simulink model "MassTransfer"  (R2023a)
settings: Solver=ode4  StartTime=0.0  StopTime=7540  FixedStep=Delta  RelTol=1e-3
values from neighbouring files (symbols this model uses):
  C2Ini = 1.6    [MassTransferModelData.m]
  C3Ini = 0    [MassTransferModelData.m]
  C4Ini = 0    [MassTransferModelData.m]
  C5Ini = 1.6    [MassTransferModelData.m]
  Delta = 5    [MassTransferModelData.m]
  F = 96485    [MassTransferModelData.m]
  NCells = 120    [MassTransferModelData.m]
  VCell = 0.4968    [MassTransferModelData.m]
  VTank = 500    [MassTransferModelData.m]
  z = 1    [MassTransferModelData.m]
undefined symbols (not defined in the file or in its folder): DiscIntNeverNeededParam
(part 2 of 3)

== system MassTransfer/Liibrary block/simulink blocks/C2Cell ==
  QCell : Inport
  CTank : Inport  Port=2
  I : Inport  Port=3
  Constant : Constant  Value=F
  Constant1 : Constant  Value=VCell
  Constant2 : Constant  Value=2
  Discrete-Time Integrator : DiscreteIntegrator  IntegratorMethod=Integration: Backward Euler  InitialCondition=C2Ini  SampleTime=-1  ICPrevOutput=DiscIntNeverNeededParam  ICPrevScaledInput=DiscIntNeverNeededParam
  Divide : Product  Inputs=*/
  Divide1 : Product  Inputs=*/
  Gain : Gain  Gain=z
  Product : Product
  Product1 : Product
  Sum : Sum  Inputs=|+-
  Sum1 : Sum  Inputs=|+-
  CCell : Outport
  wires:
  I/1 -> Divide/1
  Constant/1 -> Gain/1
  Gain/1 -> Divide/2
  Constant1/1 -> Divide1/2
  Constant2/1 -> Divide1/1
  CTank/1 -> Sum/1
  Sum/1 -> Product/2
  QCell/1 -> Product/1
  Product/1 -> Sum1/1
  Divide/1 -> Sum1/2
  Sum1/1 -> Product1/1
  Divide1/1 -> Product1/2
  Product1/1 -> Discrete-Time Integrator/1
  Discrete-Time Integrator/1 -> Sum/2, CCell/1

== system MassTransfer/Liibrary block/simulink blocks/C2Tank ==
  QTank : Inport
  CCell : Inport  Port=2
  Constant : Constant  Value=VTank
  Discrete-Time Integrator : DiscreteIntegrator  IntegratorMethod=Integration: Backward Euler  InitialCondition=C2Ini  SampleTime=-1  ICPrevOutput=DiscIntNeverNeededParam  ICPrevScaledInput=DiscIntNeverNeededParam
  Divide : Product  Inputs=*/
  Product : Product
  Scope4 : Scope
  Sum : Sum  Inputs=|+-
  CTank : Outport
  wires:
  CCell/1 -> Sum/1, Scope4/1
  Sum/1 -> Product/1
  QTank/1 -> Divide/1
  Constant/1 -> Divide/2
  Divide/1 -> Product/2
  Product/1 -> Discrete-Time Integrator/1
  Discrete-Time Integrator/1 -> Sum/2, CTank/1

== system MassTransfer/Liibrary block/simulink blocks/C3Cell ==
  QCell : Inport
  CTank : Inport  Port=2
  I : Inport  Port=3
  Constant : Constant  Value=F
  Constant1 : Constant  Value=VCell
  Constant2 : Constant  Value=2
  Discrete-Time Integrator : DiscreteIntegrator  IntegratorMethod=Integration: Backward Euler  InitialCondition=C3Ini  SampleTime=-1  ICPrevOutput=DiscIntNeverNeededParam  ICPrevScaledInput=DiscIntNeverNeededParam
  Divide : Product  Inputs=*/
  Divide1 : Product  Inputs=*/
  Gain : Gain  Gain=z
  Product : Product
  Product1 : Product
  Sum : Sum  Inputs=|+-
  Sum1 : Sum  Inputs=|++
  CCell : Outport
  wires:
  Product1/1 -> Discrete-Time Integrator/1
  Divide1/1 -> Product1/2
  Sum1/1 -> Product1/1
  Divide/1 -> Sum1/2
  Product/1 -> Sum1/1
  QCell/1 -> Product/1
  Sum/1 -> Product/2
  CTank/1 -> Sum/1
  Constant2/1 -> Divide1/1
  Constant1/1 -> Divide1/2
  Gain/1 -> Divide/2
  Constant/1 -> Gain/1
  I/1 -> Divide/1
  Discrete-Time Integrator/1 -> Sum/2, CCell/1

== system MassTransfer/Liibrary block/simulink blocks/C3Tank ==
  QTank : Inport
  CCell : Inport  Port=2
  Constant : Constant  Value=VTank
  Discrete-Time Integrator : DiscreteIntegrator  IntegratorMethod=Integration: Backward Euler  InitialCondition=C3Ini  SampleTime=-1  ICPrevOutput=DiscIntNeverNeededParam  ICPrevScaledInput=DiscIntNeverNeededParam
  Divide : Product  Inputs=*/
  Product : Product
  Sum : Sum  Inputs=|+-
  CTank : Outport
  wires:
  Product/1 -> Discrete-Time Integrator/1
  Divide/1 -> Product/2
  Constant/1 -> Divide/2
  QTank/1 -> Divide/1
  Sum/1 -> Product/1
  CCell/1 -> Sum/1
  Discrete-Time Integrator/1 -> Sum/2, CTank/1

== system MassTransfer/Liibrary block/simulink blocks/C4Cell ==
  QCell : Inport
  CTank : Inport  Port=2
  I : Inport  Port=3
  Constant : Constant  Value=F
  Constant1 : Constant  Value=VCell
  Constant2 : Constant  Value=2
  Discrete-Time Integrator : DiscreteIntegrator  IntegratorMethod=Integration: Backward Euler  InitialCondition=C4Ini  SampleTime=-1  ICPrevOutput=DiscIntNeverNeededParam  ICPrevScaledInput=DiscIntNeverNeededParam
  Divide : Product  Inputs=*/
  Divide1 : Product  Inputs=*/
  Gain : Gain  Gain=z
  Product : Product
  Product1 : Product
  Sum : Sum  Inputs=|+-
  Sum1 : Sum  Inputs=|++
  CCell : Outport
  wires:
  I/1 -> Divide/1
  Constant/1 -> Gain/1
  Gain/1 -> Divide/2
  Constant1/1 -> Divide1/2
  Constant2/1 -> Divide1/1
  CTank/1 -> Sum/1
  Sum/1 -> Product/2
  QCell/1 -> Product/1
  Product/1 -> Sum1/1
  Divide/1 -> Sum1/2
  Sum1/1 -> Product1/1
  Divide1/1 -> Product1/2
  Product1/1 -> Discrete-Time Integrator/1
  Discrete-Time Integrator/1 -> Sum/2, CCell/1

== system MassTransfer/Liibrary block/simulink blocks/C4Tank ==
  QTank : Inport
  CCell : Inport  Port=2
  Constant : Constant  Value=VTank
  Discrete-Time Integrator : DiscreteIntegrator  IntegratorMethod=Integration: Backward Euler  InitialCondition=C4Ini  SampleTime=-1  ICPrevOutput=DiscIntNeverNeededParam  ICPrevScaledInput=DiscIntNeverNeededParam
  Divide : Product  Inputs=*/
  Product : Product
  Sum : Sum  Inputs=|+-
  CTank : Outport
  wires:
  CCell/1 -> Sum/1
  Sum/1 -> Product/1
  QTank/1 -> Divide/1
  Constant/1 -> Divide/2
  Divide/1 -> Product/2
  Product/1 -> Discrete-Time Integrator/1
  Discrete-Time Integrator/1 -> Sum/2, CTank/1

== system MassTransfer/Liibrary block/simulink blocks/C5Cell ==
  QCell : Inport
  CTank : Inport  Port=2
  I : Inport  Port=3
  Constant : Constant  Value=F
  Constant1 : Constant  Value=VCell
  Constant2 : Constant  Value=2
  Discrete-Time Integrator : DiscreteIntegrator  IntegratorMethod=Integration: Backward Euler  InitialCondition=C5Ini  SampleTime=-1  ICPrevOutput=DiscIntNeverNeededParam  ICPrevScaledInput=DiscIntNeverNeededParam
  Divide : Product  Inputs=*/
  Divide1 : Product  Inputs=*/
  Gain : Gain  Gain=z
  Product : Product
  Product1 : Product
  Sum : Sum  Inputs=|+-
  Sum1 : Sum  Inputs=|+-
  CCell : Outport
  wires:
  Product1/1 -> Discrete-Time Integrator/1
  Divide1/1 -> Product1/2
  Sum1/1 -> Product1/1
  Divide/1 -> Sum1/2
  Product/1 -> Sum1/1
  QCell/1 -> Product/1
  Sum/1 -> Product/2
  CTank/1 -> Sum/1
  Constant2/1 -> Divide1/1
  Constant1/1 -> Divide1/2
  Gain/1 -> Divide/2
  Constant/1 -> Gain/1
  I/1 -> Divide/1
  Discrete-Time Integrator/1 -> Sum/2, CCell/1

== system MassTransfer/Liibrary block/simulink blocks/C5Tank ==
  QTank : Inport
  CCell : Inport  Port=2
  Constant : Constant  Value=VTank
  Discrete-Time Integrator : DiscreteIntegrator  IntegratorMethod=Integration: Backward Euler  InitialCondition=C5Ini  SampleTime=-1  ICPrevOutput=DiscIntNeverNeededParam  ICPrevScaledInput=DiscIntNeverNeededParam
  Divide : Product  Inputs=*/
  Product : Product
  Sum : Sum  Inputs=|+-
  CTank : Outport
  wires:
  Product/1 -> Discrete-Time Integrator/1
  Divide/1 -> Product/2
  Constant/1 -> Divide/2
  QTank/1 -> Divide/1
  Sum/1 -> Product/1
  CCell/1 -> Sum/1
  Discrete-Time Integrator/1 -> Sum/2, CTank/1

== system MassTransfer/QF tests/Analitical/C2Cell ==
  QCell : Inport
  CTank : Inport  Port=2
  It : Inport  Port=3
  Constant : Constant  Value=-1
  Constant1 : Constant  Value=Delta
  Constant2 : Constant
  Constant3 : Constant  Value=F
  Constant4 : Constant  Value=VCell
  MATLAB Function : MATLAB Function  TreatAsAtomicUnit=on
  Memory : Memory  InitialCondition=C2Ini
  CCell : Outport
  wires:
  Constant/1 -> MATLAB Function/8(Sign)
  Constant1/1 -> MATLAB Function/9(Delta)
  Constant2/1 -> MATLAB Function/7(Z)
  QCell/1 -> MATLAB Function/1(QCell)
  Constant3/1 -> MATLAB Function/6(F)
  Constant4/1 -> MATLAB Function/4(VCell)
  MATLAB Function/1(CCell) -> Memory/1, CCell/1
  Memory/1 -> MATLAB Function/3(CCellAnt)
  It/1 -> MATLAB Function/5(It)
  CTank/1 -> MATLAB Function/2(CTank)

== system MassTransfer/QF tests/Analitical/C2Tank ==
  QTank : Inport
  CCell : Inport  Port=2
  Constant : Constant  Value=Delta
  Constant1 : Constant  Value=VTank
  MATLAB Function : MATLAB Function  TreatAsAtomicUnit=on
  Memory : Memory  InitialCondition=C2Ini
  Scope4 : Scope
  CTank : Outport
  wires:
  Constant/1 -> MATLAB Function/5(Delta)
  Constant1/1 -> MATLAB Function/4(VTank)
  MATLAB Function/1(CTank) -> Memory/1, CTank/1
  Memory/1 -> MATLAB Function/3(CTankAnt)
  QTank/1 -> MATLAB Function/1(Q)
  CCell/1 -> Scope4/1, MATLAB Function/2(CCell)

== system MassTransfer/QF tests/Analitical/C3Cell ==
  QCell : Inport
  CTank : Inport  Port=2
  It : Inport  Port=3
  Constant : Constant
  Constant1 : Constant  Value=Delta
  Constant2 : Constant
  Constant3 : Constant  Value=F
  Constant4 : Constant  Value=VCell
  MATLAB Function : MATLAB Function  TreatAsAtomicUnit=on
  Memory : Memory  InitialCondition=C3Ini
  CCell : Outport
  wires:
  It/1 -> MATLAB Function/5(It)
  Memory/1 -> MATLAB Function/3(CCellAnt)
  MATLAB Function/1(CCell) -> Memory/1, CCell/1
  Constant4/1 -> MATLAB Function/4(VCell)
  Constant3/1 -> MATLAB Function/6(F)
  QCell/1 -> MATLAB Function/1(QCell)
  Constant2/1 -> MATLAB Function/7(Z)
  Constant1/1 -> MATLAB Function/9(Delta)
  Constant/1 -> MATLAB Function/8(Sign)
  CTank/1 -> MATLAB Function/2(CTank)

== system MassTransfer/QF tests/Analitical/C3Tank ==
  QTank : Inport
  CCell : Inport  Port=2
  Constant : Constant  Value=Delta
  Constant1 : Constant  Value=VTank
  MATLAB Function : MATLAB Function  TreatAsAtomicUnit=on
  Memory : Memory  InitialCondition=C3Ini
  CTank : Outport
  wires:
  QTank/1 -> MATLAB Function/1(Q)
  Memory/1 -> MATLAB Function/3(CTankAnt)
  MATLAB Function/1(CTank) -> Memory/1, CTank/1
  Constant1/1 -> MATLAB Function/4(VTank)
  Constant/1 -> MATLAB Function/5(Delta)
  CCell/1 -> MATLAB Function/2(CCell)

== system MassTransfer/QF tests/Analitical/C4Cell ==
  QCell : Inport
  CTank : Inport  Port=2
  It : Inport  Port=3
  Constant : Constant
  Constant1 : Constant  Value=Delta
  Constant2 : Constant
  Constant3 : Constant  Value=F
  Constant4 : Constant  Value=VCell
  MATLAB Function : MATLAB Function  TreatAsAtomicUnit=on
  Memory : Memory  InitialCondition=C4Ini
  CCell : Outport
  wires:
  Constant/1 -> MATLAB Function/8(Sign)
  Constant1/1 -> MATLAB Function/9(Delta)
  Constant2/1 -> MATLAB Function/7(Z)
  QCell/1 -> MATLAB Function/1(QCell)
  Constant3/1 -> MATLAB Function/6(F)
  Constant4/1 -> MATLAB Function/4(VCell)
  MATLAB Function/1(CCell) -> Memory/1, CCell/1
  Memory/1 -> MATLAB Function/3(CCellAnt)
  It/1 -> MATLAB Function/5(It)
  CTank/1 -> MATLAB Function/2(CTank)

== system MassTransfer/QF tests/Analitical/C4Tank ==
  QTank : Inport
  CCell : Inport  Port=2
  Constant : Constant  Value=Delta
  Constant1 : Constant  Value=VTank
  MATLAB Function : MATLAB Function  TreatAsAtomicUnit=on
  Memory : Memory  InitialCondition=C4Ini
  CTank : Outport
  wires:
  Constant/1 -> MATLAB Function/5(Delta)
  Constant1/1 -> MATLAB Function/4(VTank)
  MATLAB Function/1(CTank) -> Memory/1, CTank/1
  Memory/1 -> MATLAB Function/3(CTankAnt)
  QTank/1 -> MATLAB Function/1(Q)
  CCell/1 -> MATLAB Function/2(CCell)

== system MassTransfer/QF tests/Analitical/C5Cell ==
  QCell : Inport
  CTank : Inport  Port=2
  It : Inport  Port=3
  Constant : Constant  Value=-1
  Constant1 : Constant  Value=Delta
  Constant2 : Constant
  Constant3 : Constant  Value=F
  Constant4 : Constant  Value=VCell
  MATLAB Function : MATLAB Function  TreatAsAtomicUnit=on
  Memory : Memory  InitialCondition=C5Ini
  CCell : Outport
  wires:
  It/1 -> MATLAB Function/5(It)
  Memory/1 -> MATLAB Function/3(CCellAnt)
  MATLAB Function/1(CCell) -> Memory/1, CCell/1
  Constant4/1 -> MATLAB Function/4(VCell)
  Constant3/1 -> MATLAB Function/6(F)
  QCell/1 -> MATLAB Function/1(QCell)
  Constant2/1 -> MATLAB Function/7(Z)
  Constant1/1 -> MATLAB Function/9(Delta)
  Constant/1 -> MATLAB Function/8(Sign)
  CTank/1 -> MATLAB Function/2(CTank)

== system MassTransfer/QF tests/Analitical/C5Tank ==
  QTank : Inport
  CCell : Inport  Port=2
  Constant : Constant  Value=Delta
  Constant1 : Constant  Value=VTank
  MATLAB Function : MATLAB Function  TreatAsAtomicUnit=on
  Memory : Memory  InitialCondition=C5Ini
  Scope : Scope
  CTank : Outport
  wires:
  QTank/1 -> MATLAB Function/1(Q)
  Memory/1 -> MATLAB Function/3(CTankAnt)
  MATLAB Function/1(CTank) -> Memory/1, CTank/1
  Constant1/1 -> MATLAB Function/4(VTank)
  Constant/1 -> MATLAB Function/5(Delta)
  CCell/1 -> MATLAB Function/2(CCell), Scope/1

== system MassTransfer/QF tests1/Analitical/C2Cell ==
  QCell : Inport
  CTank : Inport  Port=2
  It : Inport  Port=3
  Constant : Constant  Value=-1
  Constant1 : Constant  Value=Delta
  Constant2 : Constant
  Constant3 : Constant  Value=F
  Constant4 : Constant  Value=VCell
  MATLAB Function : MATLAB Function  TreatAsAtomicUnit=on
  Memory : Memory  InitialCondition=C2Ini
  CCell : Outport
  wires:
  CTank/1 -> MATLAB Function/2(CTank)
  It/1 -> MATLAB Function/5(It)
  Memory/1 -> MATLAB Function/3(CCellAnt)
  MATLAB Function/1(CCell) -> CCell/1, Memory/1
  Constant4/1 -> MATLAB Function/4(VCell)
  Constant3/1 -> MATLAB Function/6(F)
  QCell/1 -> MATLAB Function/1(QCell)
  Constant2/1 -> MATLAB Function/7(Z)
  Constant1/1 -> MATLAB Function/9(Delta)
  Constant/1 -> MATLAB Function/8(Sign)

== system MassTransfer/QF tests1/Analitical/C2Tank ==
  QTank : Inport
  CCell : Inport  Port=2
  Constant : Constant  Value=Delta
  Constant1 : Constant  Value=VTank
  MATLAB Function : MATLAB Function  TreatAsAtomicUnit=on
  Memory : Memory  InitialCondition=C2Ini
  Scope4 : Scope
  CTank : Outport
  wires:
  CCell/1 -> MATLAB Function/2(CCell), Scope4/1
  QTank/1 -> MATLAB Function/1(Q)
  Memory/1 -> MATLAB Function/3(CTankAnt)
  MATLAB Function/1(CTank) -> CTank/1, Memory/1
  Constant1/1 -> MATLAB Function/4(VTank)
  Constant/1 -> MATLAB Function/5(Delta)

== system MassTransfer/QF tests1/Analitical/C3Cell ==
  QCell : Inport
  CTank : Inport  Port=2
  It : Inport  Port=3
  Constant : Constant
  Constant1 : Constant  Value=Delta
  Constant2 : Constant
  Constant3 : Constant  Value=F
  Constant4 : Constant  Value=VCell
  MATLAB Function : MATLAB Function  TreatAsAtomicUnit=on
  Memory : Memory  InitialCondition=C3Ini
  CCell : Outport
  wires:
  CTank/1 -> MATLAB Function/2(CTank)
  Constant/1 -> MATLAB Function/8(Sign)
  Constant1/1 -> MATLAB Function/9(Delta)
  Constant2/1 -> MATLAB Function/7(Z)
  QCell/1 -> MATLAB Function/1(QCell)
  Constant3/1 -> MATLAB Function/6(F)
  Constant4/1 -> MATLAB Function/4(VCell)
  MATLAB Function/1(CCell) -> CCell/1, Memory/1
  Memory/1 -> MATLAB Function/3(CCellAnt)
  It/1 -> MATLAB Function/5(It)

== system MassTransfer/QF tests1/Analitical/C3Tank ==
  QTank : Inport
  CCell : Inport  Port=2
  Constant : Constant  Value=Delta
  Constant1 : Constant  Value=VTank
  MATLAB Function : MATLAB Function  TreatAsAtomicUnit=on
  Memory : Memory  InitialCondition=C3Ini
  CTank : Outport
  wires:
  CCell/1 -> MATLAB Function/2(CCell)
  Constant/1 -> MATLAB Function/5(Delta)
  Constant1/1 -> MATLAB Function/4(VTank)
  MATLAB Function/1(CTank) -> CTank/1, Memory/1
  Memory/1 -> MATLAB Function/3(CTankAnt)
  QTank/1 -> MATLAB Function/1(Q)

== system MassTransfer/QF tests1/Analitical/C4Cell ==
  QCell : Inport
  CTank : Inport  Port=2
  It : Inport  Port=3
  Constant : Constant
  Constant1 : Constant  Value=Delta
  Constant2 : Constant
  Constant3 : Constant  Value=F
  Constant4 : Constant  Value=VCell
  MATLAB Function : MATLAB Function  TreatAsAtomicUnit=on
  Memory : Memory  InitialCondition=C4Ini
  CCell : Outport
  wires:
  CTank/1 -> MATLAB Function/2(CTank)
  It/1 -> MATLAB Function/5(It)
  Memory/1 -> MATLAB Function/3(CCellAnt)
  MATLAB Function/1(CCell) -> CCell/1, Memory/1
  Constant4/1 -> MATLAB Function/4(VCell)
  Constant3/1 -> MATLAB Function/6(F)
  QCell/1 -> MATLAB Function/1(QCell)
  Constant2/1 -> MATLAB Function/7(Z)
  Constant1/1 -> MATLAB Function/9(Delta)
  Constant/1 -> MATLAB Function/8(Sign)

== system MassTransfer/QF tests1/Analitical/C4Tank ==
  QTank : Inport
  CCell : Inport  Port=2
  Constant : Constant  Value=Delta
  Constant1 : Constant  Value=VTank
  MATLAB Function : MATLAB Function  TreatAsAtomicUnit=on
  Memory : Memory  InitialCondition=C4Ini
  CTank : Outport
  wires:
  CCell/1 -> MATLAB Function/2(CCell)
  QTank/1 -> MATLAB Function/1(Q)
  Memory/1 -> MATLAB Function/3(CTankAnt)
  MATLAB Function/1(CTank) -> CTank/1, Memory/1
  Constant1/1 -> MATLAB Function/4(VTank)
  Constant/1 -> MATLAB Function/5(Delta)

== system MassTransfer/QF tests1/Analitical/C5Cell ==
  QCell : Inport
  CTank : Inport  Port=2
  It : Inport  Port=3
  Constant : Constant  Value=-1
  Constant1 : Constant  Value=Delta
  Constant2 : Constant
  Constant3 : Constant  Value=F
  Constant4 : Constant  Value=VCell
  MATLAB Function : MATLAB Function  TreatAsAtomicUnit=on
  Memory : Memory  InitialCondition=C5Ini
  CCell : Outport
  wires:
  CTank/1 -> MATLAB Function/2(CTank)
  Constant/1 -> MATLAB Function/8(Sign)
  Constant1/1 -> MATLAB Function/9(Delta)
  Constant2/1 -> MATLAB Function/7(Z)
  QCell/1 -> MATLAB Function/1(QCell)
  Constant3/1 -> MATLAB Function/6(F)
  Constant4/1 -> MATLAB Function/4(VCell)
  MATLAB Function/1(CCell) -> CCell/1, Memory/1
  Memory/1 -> MATLAB Function/3(CCellAnt)
  It/1 -> MATLAB Function/5(It)

== system MassTransfer/QF tests1/Analitical/C5Tank ==
  QTank : Inport
  CCell : Inport  Port=2
  Constant : Constant  Value=Delta
  Constant1 : Constant  Value=VTank
  MATLAB Function : MATLAB Function  TreatAsAtomicUnit=on
  Memory : Memory  InitialCondition=C5Ini
  Scope : Scope
  CTank : Outport
  wires:
  CCell/1 -> Scope/1, MATLAB Function/2(CCell)
  Constant/1 -> MATLAB Function/5(Delta)
  Constant1/1 -> MATLAB Function/4(VTank)
  MATLAB Function/1(CTank) -> CTank/1, Memory/1
  Memory/1 -> MATLAB Function/3(CTankAnt)
  QTank/1 -> MATLAB Function/1(Q)

== system MassTransfer/QF tests3/Analitical/C2Cell ==
  QCell : Inport
  CTank : Inport  Port=2
  It : Inport  Port=3
  Constant : Constant  Value=-1
  Constant1 : Constant  Value=Delta
  Constant2 : Constant
  Constant3 : Constant  Value=F
  Constant4 : Constant  Value=VCell
  MATLAB Function : MATLAB Function  TreatAsAtomicUnit=on
  Memory : Memory  InitialCondition=C2Ini
  CCell : Outport
  wires:
  CTank/1 -> MATLAB Function/2(CTank)
  It/1 -> MATLAB Function/5(It)
  Memory/1 -> MATLAB Function/3(CCellAnt)
  MATLAB Function/1(CCell) -> CCell/1, Memory/1
  Constant4/1 -> MATLAB Function/4(VCell)
  Constant3/1 -> MATLAB Function/6(F)
  QCell/1 -> MATLAB Function/1(QCell)
  Constant2/1 -> MATLAB Function/7(Z)
  Constant1/1 -> MATLAB Function/9(Delta)
  Constant/1 -> MATLAB Function/8(Sign)

== system MassTransfer/QF tests3/Analitical/C2Tank ==
  QTank : Inport
  CCell : Inport  Port=2
  Constant : Constant  Value=Delta
  Constant1 : Constant  Value=VTank
  MATLAB Function : MATLAB Function  TreatAsAtomicUnit=on
  Memory : Memory  InitialCondition=C2Ini
  Scope4 : Scope
  CTank : Outport
  wires:
  CCell/1 -> MATLAB Function/2(CCell), Scope4/1
  QTank/1 -> MATLAB Function/1(Q)
  Memory/1 -> MATLAB Function/3(CTankAnt)
  MATLAB Function/1(CTank) -> CTank/1, Memory/1
  Constant1/1 -> MATLAB Function/4(VTank)
  Constant/1 -> MATLAB Function/5(Delta)

== system MassTransfer/QF tests3/Analitical/C3Cell ==
  QCell : Inport
  CTank : Inport  Port=2
  It : Inport  Port=3
  Constant : Constant
  Constant1 : Constant  Value=Delta
  Constant2 : Constant
  Constant3 : Constant  Value=F
  Constant4 : Constant  Value=VCell
  MATLAB Function : MATLAB Function  TreatAsAtomicUnit=on
  Memory : Memory  InitialCondition=C3Ini
  CCell : Outport
  wires:
  CTank/1 -> MATLAB Function/2(CTank)
  Constant/1 -> MATLAB Function/8(Sign)
  Constant1/1 -> MATLAB Function/9(Delta)
  Constant2/1 -> MATLAB Function/7(Z)
  QCell/1 -> MATLAB Function/1(QCell)
  Constant3/1 -> MATLAB Function/6(F)
  Constant4/1 -> MATLAB Function/4(VCell)
  MATLAB Function/1(CCell) -> CCell/1, Memory/1
  Memory/1 -> MATLAB Function/3(CCellAnt)
  It/1 -> MATLAB Function/5(It)

== system MassTransfer/QF tests3/Analitical/C3Tank ==
  QTank : Inport
  CCell : Inport  Port=2
  Constant : Constant  Value=Delta
  Constant1 : Constant  Value=VTank
  MATLAB Function : MATLAB Function  TreatAsAtomicUnit=on
  Memory : Memory  InitialCondition=C3Ini
  CTank : Outport
  wires:
  CCell/1 -> MATLAB Function/2(CCell)
  Constant/1 -> MATLAB Function/5(Delta)
  Constant1/1 -> MATLAB Function/4(VTank)
  MATLAB Function/1(CTank) -> CTank/1, Memory/1
  Memory/1 -> MATLAB Function/3(CTankAnt)
  QTank/1 -> MATLAB Function/1(Q)

== system MassTransfer/QF tests3/Analitical/C4Cell ==
  QCell : Inport
  CTank : Inport  Port=2
  It : Inport  Port=3
  Constant : Constant
  Constant1 : Constant  Value=Delta
  Constant2 : Constant
  Constant3 : Constant  Value=F
  Constant4 : Constant  Value=VCell
  MATLAB Function : MATLAB Function  TreatAsAtomicUnit=on
  Memory : Memory  InitialCondition=C4Ini
  CCell : Outport
  wires:
  CTank/1 -> MATLAB Function/2(CTank)
  It/1 -> MATLAB Function/5(It)
  Memory/1 -> MATLAB Function/3(CCellAnt)
  MATLAB Function/1(CCell) -> CCell/1, Memory/1
  Constant4/1 -> MATLAB Function/4(VCell)
  Constant3/1 -> MATLAB Function/6(F)
  QCell/1 -> MATLAB Function/1(QCell)
  Constant2/1 -> MATLAB Function/7(Z)
  Constant1/1 -> MATLAB Function/9(Delta)
  Constant/1 -> MATLAB Function/8(Sign)

== system MassTransfer/QF tests3/Analitical/C4Tank ==
  QTank : Inport
  CCell : Inport  Port=2
  Constant : Constant  Value=Delta
  Constant1 : Constant  Value=VTank
  MATLAB Function : MATLAB Function  TreatAsAtomicUnit=on
  Memory : Memory  InitialCondition=C4Ini
  CTank : Outport
  wires:
  CCell/1 -> MATLAB Function/2(CCell)
  QTank/1 -> MATLAB Function/1(Q)
  Memory/1 -> MATLAB Function/3(CTankAnt)
  MATLAB Function/1(CTank) -> CTank/1, Memory/1
  Constant1/1 -> MATLAB Function/4(VTank)
  Constant/1 -> MATLAB Function/5(Delta)

== system MassTransfer/QF tests3/Analitical/C5Cell ==
  QCell : Inport
  CTank : Inport  Port=2
  It : Inport  Port=3
  Constant : Constant  Value=-1
  Constant1 : Constant  Value=Delta
  Constant2 : Constant
  Constant3 : Constant  Value=F
  Constant4 : Constant  Value=VCell
  MATLAB Function : MATLAB Function  TreatAsAtomicUnit=on
  Memory : Memory  InitialCondition=C5Ini
  CCell : Outport
  wires:
  CTank/1 -> MATLAB Function/2(CTank)
  Constant/1 -> MATLAB Function/8(Sign)
  Constant1/1 -> MATLAB Function/9(Delta)
  Constant2/1 -> MATLAB Function/7(Z)
  QCell/1 -> MATLAB Function/1(QCell)
  Constant3/1 -> MATLAB Function/6(F)
  Constant4/1 -> MATLAB Function/4(VCell)
  MATLAB Function/1(CCell) -> CCell/1, Memory/1
  Memory/1 -> MATLAB Function/3(CCellAnt)
  It/1 -> MATLAB Function/5(It)

== system MassTransfer/QF tests3/Analitical/C5Tank ==
  QTank : Inport
  CCell : Inport  Port=2
  Constant : Constant  Value=Delta
  Constant1 : Constant  Value=VTank
  MATLAB Function : MATLAB Function  TreatAsAtomicUnit=on
  Memory : Memory  InitialCondition=C5Ini
  Scope : Scope
  CTank : Outport
  wires:
  CCell/1 -> Scope/1, MATLAB Function/2(CCell)
  Constant/1 -> MATLAB Function/5(Delta)
  Constant1/1 -> MATLAB Function/4(VTank)
  MATLAB Function/1(CTank) -> CTank/1, Memory/1
  Memory/1 -> MATLAB Function/3(CTankAnt)
  QTank/1 -> MATLAB Function/1(Q)

== system MassTransfer/QF tests4/ Sim /C2Cell ==
  QCell : Inport
  C2Tank : Inport  Port=2
  Cr : Inport  Port=3
  Qf : Inport  Port=4
  Sign : Inport  Port=5
  Constant4 : Constant  Value=VCell
  Constant5 : Constant  Value=2
  Discrete-Time Integrator : DiscreteIntegrator  IntegratorMethod=Integration: Backward Euler  InitialCondition=C2Ini  SampleTime=-1  ICPrevOutput=DiscIntNeverNeededParam  ICPrevScaledInput=DiscIntNeverNeededParam
  Divide : Product  Inputs=*/
  Divide1 : Product  Inputs=*/
  Product : Product
  Product1 : Product
  Product2 : Product
  Sum : Sum  Inputs=|+-
  Sum1 : Sum  Inputs=|+-
  C2Cell : Outport
  wires:
  Product1/1 -> Discrete-Time Integrator/1
  Sum1/1 -> Product1/1
  Product2/1 -> Sum1/2
  Sum/1 -> Sum1/1
  Sign/1 -> Product2/1
  Divide1/1 -> Product2/2
  Qf/1 -> Divide1/2
  Cr/1 -> Divide1/1
  Product/1 -> Product1/2
  Discrete-Time Integrator/1 -> Sum/2, C2Cell/1
  QCell/1 -> Product/1
  Divide/1 -> Product/2
  C2Tank/1 -> Sum/1
  Constant5/1 -> Divide/1
  Constant4/1 -> Divide/2

== system MassTransfer/QF tests4/ Sim /C2Tank ==
  QTank : Inport
  C2Cell : Inport  Port=2
  Constant : Constant  Value=VTank
  Discrete-Time Integrator : DiscreteIntegrator  IntegratorMethod=Integration: Backward Euler  InitialCondition=C2Ini  SampleTime=-1  ICPrevOutput=DiscIntNeverNeededParam  ICPrevScaledInput=DiscIntNeverNeededParam
  Divide : Product  Inputs=*/
  Product : Product
  Sum : Sum  Inputs=|+-
  C2Tank : Outport
  wires:
  Discrete-Time Integrator/1 -> Sum/2, C2Tank/1
  Product/1 -> Discrete-Time Integrator/1
  Divide/1 -> Product/2
  Constant/1 -> Divide/2
  QTank/1 -> Divide/1
  Sum/1 -> Product/1
  C2Cell/1 -> Sum/1

== system MassTransfer/QF tests4/ Sim /C3Cell ==
  QCell : Inport
  C3Tank : Inport  Port=2
  Cr : Inport  Port=3
  Qf : Inport  Port=4
  Sign : Inport  Port=5
  Constant4 : Constant  Value=VCell
  Constant5 : Constant  Value=2
  Discrete-Time Integrator : DiscreteIntegrator  IntegratorMethod=Integration: Backward Euler  InitialCondition=C3Ini  SampleTime=-1  ICPrevOutput=DiscIntNeverNeededParam  ICPrevScaledInput=DiscIntNeverNeededParam
  Divide : Product  Inputs=*/
  Divide1 : Product  Inputs=*/
  Product : Product
  Product1 : Product
  Product2 : Product
  Sum : Sum  Inputs=|+-
  Sum1 : Sum  Inputs=|++
  C3Cell : Outport
  wires:
  Constant4/1 -> Divide/2
  Constant5/1 -> Divide/1
  C3Tank/1 -> Sum/1
  Divide/1 -> Product/2
  QCell/1 -> Product/1
  Discrete-Time Integrator/1 -> C3Cell/1, Sum/2
  Product/1 -> Product1/2
  Cr/1 -> Divide1/1
  Qf/1 -> Divide1/2
  Divide1/1 -> Product2/2
  Sign/1 -> Product2/1
  Sum/1 -> Sum1/1
  Product2/1 -> Sum1/2
  Sum1/1 -> Product1/1
  Product1/1 -> Discrete-Time Integrator/1

== system MassTransfer/QF tests4/ Sim /C3Tank ==
  QTank : Inport
  C3Cell : Inport  Port=2
  Constant : Constant  Value=VTank
  Discrete-Time Integrator : DiscreteIntegrator  IntegratorMethod=Integration: Backward Euler  InitialCondition=C3Ini  SampleTime=-1  ICPrevOutput=DiscIntNeverNeededParam  ICPrevScaledInput=DiscIntNeverNeededParam
  Divide : Product  Inputs=*/
  Product : Product
  Sum : Sum  Inputs=|+-
  C3Tank : Outport
  wires:
  Discrete-Time Integrator/1 -> Sum/2, C3Tank/1
  C3Cell/1 -> Sum/1
  Sum/1 -> Product/1
  QTank/1 -> Divide/1
  Constant/1 -> Divide/2
  Divide/1 -> Product/2
  Product/1 -> Discrete-Time Integrator/1

== system MassTransfer/QF tests4/ Sim /C4Cell ==
  QCell : Inport
  C4Tank : Inport  Port=2
  Cr : Inport  Port=3
  Qf : Inport  Port=4
  Sign : Inport  Port=5
  Constant4 : Constant  Value=VCell
  Constant5 : Constant  Value=2
  Discrete-Time Integrator : DiscreteIntegrator  IntegratorMethod=Integration: Backward Euler  InitialCondition=C4Ini  SampleTime=-1  ICPrevOutput=DiscIntNeverNeededParam  ICPrevScaledInput=DiscIntNeverNeededParam
  Divide : Product  Inputs=*/
  Divide1 : Product  Inputs=*/
  Product : Product
  Product1 : Product
  Product2 : Product
  Sum : Sum  Inputs=|+-
  Sum1 : Sum  Inputs=|++
  C4Cell : Outport
  wires:
  Product1/1 -> Discrete-Time Integrator/1
  Sum1/1 -> Product1/1
  Product2/1 -> Sum1/2
  Sum/1 -> Sum1/1
  Sign/1 -> Product2/1
  Divide1/1 -> Product2/2
  Qf/1 -> Divide1/2
  Cr/1 -> Divide1/1
  Product/1 -> Product1/2
  Discrete-Time Integrator/1 -> Sum/2, C4Cell/1
  QCell/1 -> Product/1
  Divide/1 -> Product/2
  C4Tank/1 -> Sum/1
  Constant5/1 -> Divide/1
  Constant4/1 -> Divide/2

== system MassTransfer/QF tests4/ Sim /C4Cell1 ==
  QCell : Inport
  C5Tank : Inport  Port=2
  Cr : Inport  Port=3
  Qf : Inport  Port=4
  Sign : Inport  Port=5
  Constant4 : Constant  Value=VCell
  Constant5 : Constant  Value=2
  Discrete-Time Integrator : DiscreteIntegrator  IntegratorMethod=Integration: Backward Euler  InitialCondition=C5Ini  SampleTime=-1  ICPrevOutput=DiscIntNeverNeededParam  ICPrevScaledInput=DiscIntNeverNeededParam
  Divide : Product  Inputs=*/
  Divide1 : Product  Inputs=*/
  Product : Product
  Product1 : Product
  Product2 : Product
  Sum : Sum  Inputs=|+-
  Sum1 : Sum  Inputs=|+-
  C5Cell : Outport
  wires:
  Constant4/1 -> Divide/2
  Constant5/1 -> Divide/1
  C5Tank/1 -> Sum/1
  Divide/1 -> Product/2
  QCell/1 -> Product/1
  Discrete-Time Integrator/1 -> C5Cell/1, Sum/2
  Product/1 -> Product1/2
  Cr/1 -> Divide1/1
  Qf/1 -> Divide1/2
  Divide1/1 -> Product2/2
  Sign/1 -> Product2/1
  Sum/1 -> Sum1/1
  Product2/1 -> Sum1/2
  Sum1/1 -> Product1/1
  Product1/1 -> Discrete-Time Integrator/1

== system MassTransfer/QF tests4/ Sim /C4Tank ==
  QTank : Inport
  C4Cell : Inport  Port=2
  Constant : Constant  Value=VTank
  Discrete-Time Integrator : DiscreteIntegrator  IntegratorMethod=Integration: Backward Euler  InitialCondition=C4Ini  SampleTime=-1  ICPrevOutput=DiscIntNeverNeededParam  ICPrevScaledInput=DiscIntNeverNeededParam
  Divide : Product  Inputs=*/
  Product : Product
  Sum : Sum  Inputs=|+-
  C4Tank : Outport
  wires:
  Discrete-Time Integrator/1 -> C4Tank/1, Sum/2
  Product/1 -> Discrete-Time Integrator/1
  Divide/1 -> Product/2
  Constant/1 -> Divide/2
  QTank/1 -> Divide/1
  Sum/1 -> Product/1
  C4Cell/1 -> Sum/1

== system MassTransfer/QF tests4/ Sim /C5Tank ==
  QTank : Inport
  C5Cell : Inport  Port=2
  Constant : Constant  Value=VTank
  Discrete-Time Integrator : DiscreteIntegrator  IntegratorMethod=Integration: Backward Euler  InitialCondition=C5Ini  SampleTime=-1  ICPrevOutput=DiscIntNeverNeededParam  ICPrevScaledInput=DiscIntNeverNeededParam
  Divide : Product  Inputs=*/
  Product : Product
  Sum : Sum  Inputs=|+-
  C5Tank : Outport
  wires:
  Discrete-Time Integrator/1 -> Sum/2, C5Tank/1
  C5Cell/1 -> Sum/1
  Sum/1 -> Product/1
  QTank/1 -> Divide/1
  Constant/1 -> Divide/2
  Divide/1 -> Product/2
  Product/1 -> Discrete-Time Integrator/1

== system MassTransfer/QF tests5/ Sim /C2Cell ==
  QCell : Inport
  C2Tank : Inport  Port=2
  Cr : Inport  Port=3
  Qf : Inport  Port=4
  Sign : Inport  Port=5
  Constant4 : Constant  Value=VCell
  Constant5 : Constant  Value=2
  Discrete-Time Integrator : DiscreteIntegrator  IntegratorMethod=Integration: Backward Euler  InitialCondition=C2Ini  SampleTime=-1  ICPrevOutput=DiscIntNeverNeededParam  ICPrevScaledInput=DiscIntNeverNeededParam
  Divide : Product  Inputs=*/
  Divide1 : Product  Inputs=*/
  Product : Product
  Product1 : Product
  Product2 : Product
  Sum : Sum  Inputs=|+-
  Sum1 : Sum  Inputs=|+-
  C2Cell : Outport
  wires:
  Constant4/1 -> Divide/2
  Constant5/1 -> Divide/1
  C2Tank/1 -> Sum/1
  Divide/1 -> Product/2
  QCell/1 -> Product/1
  Discrete-Time Integrator/1 -> C2Cell/1, Sum/2
  Product/1 -> Product1/2
  Cr/1 -> Divide1/1
  Qf/1 -> Divide1/2
  Divide1/1 -> Product2/2
  Sign/1 -> Product2/1
  Sum/1 -> Sum1/1
  Product2/1 -> Sum1/2
  Sum1/1 -> Product1/1
  Product1/1 -> Discrete-Time Integrator/1

== system MassTransfer/QF tests5/ Sim /C2Tank ==
  QTank : Inport
  C2Cell : Inport  Port=2
  Constant : Constant  Value=VTank
  Discrete-Time Integrator : DiscreteIntegrator  IntegratorMethod=Integration: Backward Euler  InitialCondition=C2Ini  SampleTime=-1  ICPrevOutput=DiscIntNeverNeededParam  ICPrevScaledInput=DiscIntNeverNeededParam
  Divide : Product  Inputs=*/
  Product : Product
  Sum : Sum  Inputs=|+-
  C2Tank : Outport
  wires:
  C2Cell/1 -> Sum/1
  Sum/1 -> Product/1
  QTank/1 -> Divide/1
  Constant/1 -> Divide/2
  Divide/1 -> Product/2
  Product/1 -> Discrete-Time Integrator/1
  Discrete-Time Integrator/1 -> C2Tank/1, Sum/2

== system MassTransfer/QF tests5/ Sim /C3Cell ==
  QCell : Inport
  C3Tank : Inport  Port=2
  Cr : Inport  Port=3
  Qf : Inport  Port=4
  Sign : Inport  Port=5
  Constant4 : Constant  Value=VCell
  Constant5 : Constant  Value=2
  Discrete-Time Integrator : DiscreteIntegrator  IntegratorMethod=Integration: Backward Euler  InitialCondition=C3Ini  SampleTime=-1  ICPrevOutput=DiscIntNeverNeededParam  ICPrevScaledInput=DiscIntNeverNeededParam
  Divide : Product  Inputs=*/
  Divide1 : Product  Inputs=*/
  Product : Product
  Product1 : Product
  Product2 : Product
  Sum : Sum  Inputs=|+-
  Sum1 : Sum  Inputs=|++
  C3Cell : Outport
  wires:
  Product1/1 -> Discrete-Time Integrator/1
  Sum1/1 -> Product1/1
  Product2/1 -> Sum1/2
  Sum/1 -> Sum1/1
  Sign/1 -> Product2/1
  Divide1/1 -> Product2/2
  Qf/1 -> Divide1/2
  Cr/1 -> Divide1/1
  Product/1 -> Product1/2
  Discrete-Time Integrator/1 -> Sum/2, C3Cell/1
  QCell/1 -> Product/1
  Divide/1 -> Product/2
  C3Tank/1 -> Sum/1
  Constant5/1 -> Divide/1
  Constant4/1 -> Divide/2

== system MassTransfer/QF tests5/ Sim /C3Tank ==
  QTank : Inport
  C3Cell : Inport  Port=2
  Constant : Constant  Value=VTank
  Discrete-Time Integrator : DiscreteIntegrator  IntegratorMethod=Integration: Backward Euler  InitialCondition=C3Ini  SampleTime=-1  ICPrevOutput=DiscIntNeverNeededParam  ICPrevScaledInput=DiscIntNeverNeededParam
  Divide : Product  Inputs=*/
  Product : Product
  Sum : Sum  Inputs=|+-
  C3Tank : Outport
  wires:
  Product/1 -> Discrete-Time Integrator/1
  Divide/1 -> Product/2
  Constant/1 -> Divide/2
  QTank/1 -> Divide/1
  Sum/1 -> Product/1
  C3Cell/1 -> Sum/1
  Discrete-Time Integrator/1 -> C3Tank/1, Sum/2

== system MassTransfer/QF tests5/ Sim /C4Cell ==
  QCell : Inport
  C4Tank : Inport  Port=2
  Cr : Inport  Port=3
  Qf : Inport  Port=4
  Sign : Inport  Port=5
  Constant4 : Constant  Value=VCell
  Constant5 : Constant  Value=2
  Discrete-Time Integrator : DiscreteIntegrator  IntegratorMethod=Integration: Backward Euler  InitialCondition=C4Ini  SampleTime=-1  ICPrevOutput=DiscIntNeverNeededParam  ICPrevScaledInput=DiscIntNeverNeededParam
  Divide : Product  Inputs=*/
  Divide1 : Product  Inputs=*/
  Product : Product
  Product1 : Product
  Product2 : Product
  Sum : Sum  Inputs=|+-
  Sum1 : Sum  Inputs=|++
  C4Cell : Outport
  wires:
  Constant4/1 -> Divide/2
  Constant5/1 -> Divide/1
  C4Tank/1 -> Sum/1
  Divide/1 -> Product/2
  QCell/1 -> Product/1
  Discrete-Time Integrator/1 -> C4Cell/1, Sum/2
  Product/1 -> Product1/2
  Cr/1 -> Divide1/1
  Qf/1 -> Divide1/2
  Divide1/1 -> Product2/2
  Sign/1 -> Product2/1
  Sum/1 -> Sum1/1
  Product2/1 -> Sum1/2
  Sum1/1 -> Product1/1
  Product1/1 -> Discrete-Time Integrator/1

== system MassTransfer/QF tests5/ Sim /C4Cell1 ==
  QCell : Inport
  C5Tank : Inport  Port=2
  Cr : Inport  Port=3
  Qf : Inport  Port=4
  Sign : Inport  Port=5
  Constant4 : Constant  Value=VCell
  Constant5 : Constant  Value=2
  Discrete-Time Integrator : DiscreteIntegrator  IntegratorMethod=Integration: Backward Euler  InitialCondition=C5Ini  SampleTime=-1  ICPrevOutput=DiscIntNeverNeededParam  ICPrevScaledInput=DiscIntNeverNeededParam
  Divide : Product  Inputs=*/
  Divide1 : Product  Inputs=*/
  Product : Product
  Product1 : Product
  Product2 : Product
  Sum : Sum  Inputs=|+-
  Sum1 : Sum  Inputs=|+-
  C5Cell : Outport
  wires:
  Product1/1 -> Discrete-Time Integrator/1
  Sum1/1 -> Product1/1
  Product2/1 -> Sum1/2
  Sum/1 -> Sum1/1
  Sign/1 -> Product2/1
  Divide1/1 -> Product2/2
  Qf/1 -> Divide1/2
  Cr/1 -> Divide1/1
  Product/1 -> Product1/2
  Discrete-Time Integrator/1 -> Sum/2, C5Cell/1
  QCell/1 -> Product/1
  Divide/1 -> Product/2
  C5Tank/1 -> Sum/1
  Constant5/1 -> Divide/1
  Constant4/1 -> Divide/2

== system MassTransfer/QF tests5/ Sim /C4Tank ==
  QTank : Inport
  C4Cell : Inport  Port=2
  Constant : Constant  Value=VTank
  Discrete-Time Integrator : DiscreteIntegrator  IntegratorMethod=Integration: Backward Euler  InitialCondition=C4Ini  SampleTime=-1  ICPrevOutput=DiscIntNeverNeededParam  ICPrevScaledInput=DiscIntNeverNeededParam
  Divide : Product  Inputs=*/
  Product : Product
  Sum : Sum  Inputs=|+-
  C4Tank : Outport
  wires:
  C4Cell/1 -> Sum/1
  Sum/1 -> Product/1
  QTank/1 -> Divide/1
  Constant/1 -> Divide/2
  Divide/1 -> Product/2
  Product/1 -> Discrete-Time Integrator/1
  Discrete-Time Integrator/1 -> Sum/2, C4Tank/1

== system MassTransfer/QF tests5/ Sim /C5Tank ==
  QTank : Inport
  C5Cell : Inport  Port=2
  Constant : Constant  Value=VTank
  Discrete-Time Integrator : DiscreteIntegrator  IntegratorMethod=Integration: Backward Euler  InitialCondition=C5Ini  SampleTime=-1  ICPrevOutput=DiscIntNeverNeededParam  ICPrevScaledInput=DiscIntNeverNeededParam
  Divide : Product  Inputs=*/
  Product : Product
  Sum : Sum  Inputs=|+-
  C5Tank : Outport
  wires:
  Product/1 -> Discrete-Time Integrator/1
  Divide/1 -> Product/2
  Constant/1 -> Divide/2
  QTank/1 -> Divide/1
  Sum/1 -> Product/1
  C5Cell/1 -> Sum/1
  Discrete-Time Integrator/1 -> C5Tank/1, Sum/2

== system MassTransfer/Library block sustituyendo I//(zF) en las ecuaciones/QF tests2/Simulink I//(zf) Cambiado/C2Cell ==
  QCell : Inport
  C2Tank : Inport  Port=2
  Cr : Inport  Port=3
  Qf : Inport  Port=4
  Sign : Inport  Port=5
  Constant4 : Constant  Value=VCell
  Constant5 : Constant  Value=2
  Discrete-Time Integrator : DiscreteIntegrator  IntegratorMethod=Integration: Backward Euler  InitialCondition=C2Ini  SampleTime=-1  ICPrevOutput=DiscIntNeverNeededParam  ICPrevScaledInput=DiscIntNeverNeededParam
  Divide : Product  Inputs=*/
  Divide1 : Product  Inputs=*/
  Product : Product
  Product1 : Product
  Product2 : Product
  Sum : Sum  Inputs=|+-
  Sum1 : Sum  Inputs=|+-
  C2Cell : Outport
  wires:
  Constant4/1 -> Divide/2
  Constant5/1 -> Divide/1
  C2Tank/1 -> Sum/1
  Divide/1 -> Product/2
  QCell/1 -> Product/1
  Discrete-Time Integrator/1 -> C2Cell/1, Sum/2
  Product/1 -> Product1/2
  Cr/1 -> Divide1/1
  Qf/1 -> Divide1/2
  Divide1/1 -> Product2/2
  Sign/1 -> Product2/1
  Sum/1 -> Sum1/1
  Product2/1 -> Sum1/2
  Sum1/1 -> Product1/1
  Product1/1 -> Discrete-Time Integrator/1

== system MassTransfer/Library block sustituyendo I//(zF) en las ecuaciones/QF tests2/Simulink I//(zf) Cambiado/C2Tank ==
  QTank : Inport
  C2Cell : Inport  Port=2
  Constant : Constant  Value=VTank
  Discrete-Time Integrator : DiscreteIntegrator  IntegratorMethod=Integration: Backward Euler  InitialCondition=C2Ini  SampleTime=-1  ICPrevOutput=DiscIntNeverNeededParam  ICPrevScaledInput=DiscIntNeverNeededParam
  Divide : Product  Inputs=*/
  Product : Product
  Sum : Sum  Inputs=|+-
  C2Tank : Outport
  wires:
  C2Cell/1 -> Sum/1
  Sum/1 -> Product/1
  QTank/1 -> Divide/1
  Constant/1 -> Divide/2
  Divide/1 -> Product/2
  Product/1 -> Discrete-Time Integrator/1
  Discrete-Time Integrator/1 -> C2Tank/1, Sum/2

== system MassTransfer/Library block sustituyendo I//(zF) en las ecuaciones/QF tests2/Simulink I//(zf) Cambiado/C3Cell ==
  QCell : Inport
  C3Tank : Inport  Port=2
  Cr : Inport  Port=3
  Qf : Inport  Port=4
  Sign : Inport  Port=5
  Constant4 : Constant  Value=VCell
  Constant5 : Constant  Value=2
  Discrete-Time Integrator : DiscreteIntegrator  IntegratorMethod=Integration: Backward Euler  InitialCondition=C3Ini  SampleTime=-1  ICPrevOutput=DiscIntNeverNeededParam  ICPrevScaledInput=DiscIntNeverNeededParam
  Divide : Product  Inputs=*/
  Divide1 : Product  Inputs=*/
  Product : Product
  Product1 : Product
  Product2 : Product
  Sum : Sum  Inputs=|+-
  Sum1 : Sum  Inputs=|++
  C3Cell : Outport
  wires:
  Product1/1 -> Discrete-Time Integrator/1
  Sum1/1 -> Product1/1
  Product2/1 -> Sum1/2
  Sum/1 -> Sum1/1
  Sign/1 -> Product2/1
  Divide1/1 -> Product2/2
  Qf/1 -> Divide1/2
  Cr/1 -> Divide1/1
  Product/1 -> Product1/2
  Discrete-Time Integrator/1 -> Sum/2, C3Cell/1
  QCell/1 -> Product/1
  Divide/1 -> Product/2
  C3Tank/1 -> Sum/1
  Constant5/1 -> Divide/1
  Constant4/1 -> Divide/2

== system MassTransfer/Library block sustituyendo I//(zF) en las ecuaciones/QF tests2/Simulink I//(zf) Cambiado/C3Tank ==
  QTank : Inport
  C3Cell : Inport  Port=2
  Constant : Constant  Value=VTank
  Discrete-Time Integrator : DiscreteIntegrator  IntegratorMethod=Integration: Backward Euler  InitialCondition=C3Ini  SampleTime=-1  ICPrevOutput=DiscIntNeverNeededParam  ICPrevScaledInput=DiscIntNeverNeededParam
  Divide : Product  Inputs=*/
  Product : Product
  Sum : Sum  Inputs=|+-
  C3Tank : Outport
  wires:
  Product/1 -> Discrete-Time Integrator/1
  Divide/1 -> Product/2
  Constant/1 -> Divide/2
  QTank/1 -> Divide/1
  Sum/1 -> Product/1
  C3Cell/1 -> Sum/1
  Discrete-Time Integrator/1 -> C3Tank/1, Sum/2

== system MassTransfer/Library block sustituyendo I//(zF) en las ecuaciones/QF tests2/Simulink I//(zf) Cambiado/C4Cell ==
  QCell : Inport
  C4Tank : Inport  Port=2
  Cr : Inport  Port=3
  Qf : Inport  Port=4
  Sign : Inport  Port=5
  Constant4 : Constant  Value=VCell
  Constant5 : Constant  Value=2
  Discrete-Time Integrator : DiscreteIntegrator  IntegratorMethod=Integration: Backward Euler  InitialCondition=C4Ini  SampleTime=-1  ICPrevOutput=DiscIntNeverNeededParam  ICPrevScaledInput=DiscIntNeverNeededParam
  Divide : Product  Inputs=*/
  Divide1 : Product  Inputs=*/
  Product : Product
  Product1 : Product
  Product2 : Product
  Sum : Sum  Inputs=|+-
  Sum1 : Sum  Inputs=|++
  C4Cell : Outport
  wires:
  Constant4/1 -> Divide/2
  Constant5/1 -> Divide/1
  C4Tank/1 -> Sum/1
  Divide/1 -> Product/2
  QCell/1 -> Product/1
  Discrete-Time Integrator/1 -> C4Cell/1, Sum/2
  Product/1 -> Product1/2
  Cr/1 -> Divide1/1
  Qf/1 -> Divide1/2
  Divide1/1 -> Product2/2
  Sign/1 -> Product2/1
  Sum/1 -> Sum1/1
  Product2/1 -> Sum1/2
  Sum1/1 -> Product1/1
  Product1/1 -> Discrete-Time Integrator/1

== system MassTransfer/Library block sustituyendo I//(zF) en las ecuaciones/QF tests2/Simulink I//(zf) Cambiado/C4Cell1 ==
  QCell : Inport
  C5Tank : Inport  Port=2
  Cr : Inport  Port=3
  Qf : Inport  Port=4
  Sign : Inport  Port=5
  Constant4 : Constant  Value=VCell
  Constant5 : Constant  Value=2
  Discrete-Time Integrator : DiscreteIntegrator  IntegratorMethod=Integration: Backward Euler  InitialCondition=C5Ini  SampleTime=-1  ICPrevOutput=DiscIntNeverNeededParam  ICPrevScaledInput=DiscIntNeverNeededParam
  Divide : Product  Inputs=*/
  Divide1 : Product  Inputs=*/
  Product : Product
  Product1 : Product
  Product2 : Product
  Sum : Sum  Inputs=|+-
  Sum1 : Sum  Inputs=|+-
  C5Cell : Outport
  wires:
  Product1/1 -> Discrete-Time Integrator/1
  Sum1/1 -> Product1/1
  Product2/1 -> Sum1/2
  Sum/1 -> Sum1/1
  Sign/1 -> Product2/1
  Divide1/1 -> Product2/2
  Qf/1 -> Divide1/2
  Cr/1 -> Divide1/1
  Product/1 -> Product1/2
  Discrete-Time Integrator/1 -> Sum/2, C5Cell/1
  QCell/1 -> Product/1
  Divide/1 -> Product/2
  C5Tank/1 -> Sum/1
  Constant5/1 -> Divide/1
  Constant4/1 -> Divide/2

== system MassTransfer/Library block sustituyendo I//(zF) en las ecuaciones/QF tests2/Simulink I//(zf) Cambiado/C4Tank ==
  QTank : Inport
  C4Cell : Inport  Port=2
  Constant : Constant  Value=VTank
  Discrete-Time Integrator : DiscreteIntegrator  IntegratorMethod=Integration: Backward Euler  InitialCondition=C4Ini  SampleTime=-1  ICPrevOutput=DiscIntNeverNeededParam  ICPrevScaledInput=DiscIntNeverNeededParam
  Divide : Product  Inputs=*/
  Product : Product
  Sum : Sum  Inputs=|+-
  C4Tank : Outport
  wires:
  C4Cell/1 -> Sum/1
  Sum/1 -> Product/1
  QTank/1 -> Divide/1
  Constant/1 -> Divide/2
  Divide/1 -> Product/2
  Product/1 -> Discrete-Time Integrator/1
  Discrete-Time Integrator/1 -> Sum/2, C4Tank/1

== system MassTransfer/Library block sustituyendo I//(zF) en las ecuaciones/QF tests2/Simulink I//(zf) Cambiado/C5Tank ==
  QTank : Inport
  C5Cell : Inport  Port=2
  Constant : Constant  Value=VTank
  Discrete-Time Integrator : DiscreteIntegrator  IntegratorMethod=Integration: Backward Euler  InitialCondition=C5Ini  SampleTime=-1  ICPrevOutput=DiscIntNeverNeededParam  ICPrevScaledInput=DiscIntNeverNeededParam
  Divide : Product  Inputs=*/
  Product : Product
  Sum : Sum  Inputs=|+-
  C5Tank : Outport
  wires:
  Product/1 -> Discrete-Time Integrator/1
  Divide/1 -> Product/2
  Constant/1 -> Divide/2
  QTank/1 -> Divide/1
  Sum/1 -> Product/1
  C5Cell/1 -> Sum/1
  Discrete-Time Integrator/1 -> C5Tank/1, Sum/2

== matlab function MassTransfer/QF tests/Analitical/C3Tank/MATLAB Function ==
  data: Q input; CTank output; CCell input; CTankAnt input; VTank input; Delta input
function CTank = fcn(Q, CCell, CTankAnt, VTank, Delta)
    K3 = Q/VTank;
    CTank = (CCell*K3*Delta + CTankAnt)/(1+K3*Delta);
end

== matlab function MassTransfer/QF tests/Analitical/C4Tank/MATLAB Function ==
  data: Q input; CTank output; CCell input; CTankAnt input; VTank input; Delta input
function CTank = fcn(Q, CCell, CTankAnt, VTank, Delta)
    K3 = Q/VTank;
    CTank = (CCell*K3*Delta + CTankAnt)/(1+K3*Delta);
end

== matlab function MassTransfer/QF tests/Analitical/C5Tank/MATLAB Function ==
  data: Q input; CTank output; CCell input; CTankAnt input; VTank input; Delta input
function CTank = fcn(Q, CCell, CTankAnt, VTank, Delta)
    K3 = Q/VTank;
    CTank = (CCell*K3*Delta + CTankAnt)/(1+K3*Delta);
end

== matlab function MassTransfer/QF tests/Flow calculation anal/MATLAB Function ==
  data: C2 input; QCell output; C3 input; C4 input; C5 input; I input; F input; QF input
function QCell = fcn(C2, C3, C4, C5, I, F, QF)
    if I > 0
        QCell = QF*abs(I)/(F*(C2+C5)/2);
    else
        QCell = QF*abs(I)/(F*(C3+C4)/2);
    end
end

== matlab function MassTransfer/Liibrary block/Analitical/C2Tank/MATLAB Function ==
  data: Q input; CTank output; CCell input; CTankAnt input; VTank input; Delta input
function CTank = fcn(Q, CCell, CTankAnt, VTank, Delta)
    K3 = Q/VTank;
    CTank = (CCell*K3*Delta + CTankAnt)/(1+K3*Delta);
end

== matlab function MassTransfer/Liibrary block/Analitical/C2Cell/MATLAB Function ==
  data: QCell input; CCell output; CTank input; CCellAnt input; VCell input; It input; F input; Z input; Sign input; Delta input
function CCell = fcn(QCell, CTank, CCellAnt, VCell, It, F, Z, Sign, Delta)
    K1 = QCell*(1/(VCell/2));
    K2 = (1/(VCell/2))*(1/(Z*F));
    CCell = (K1*Delta*CTank + Sign*K2*Delta*It + CCellAnt)/(1+K1*Delta);
end

== matlab function MassTransfer/Liibrary block/Analitical/C3Cell/MATLAB Function ==
  data: QCell input; CCell output; CTank input; CCellAnt input; VCell input; It input; F input; Z input; Sign input; Delta input
function CCell = fcn(QCell, CTank, CCellAnt, VCell, It, F, Z, Sign, Delta)
    K1 = QCell*(1/(VCell/2));
    K2 = (1/(VCell/2))*(1/(Z*F));
    CCell = (K1*Delta*CTank + Sign*K2*Delta*It + CCellAnt)/(1+K1*Delta);
end

== matlab function MassTransfer/Liibrary block/Analitical/C3Tank/MATLAB Function ==
  data: Q input; CTank output; CCell input; CTankAnt input; VTank input; Delta input
function CTank = fcn(Q, CCell, CTankAnt, VTank, Delta)
    K3 = Q/VTank;
    CTank = (CCell*K3*Delta + CTankAnt)/(1+K3*Delta);
end

== matlab function MassTransfer/Liibrary block/Analitical/C4Cell/MATLAB Function ==
  data: QCell input; CCell output; CTank input; CCellAnt input; VCell input; It input; F input; Z input; Sign input; Delta input
function CCell = fcn(QCell, CTank, CCellAnt, VCell, It, F, Z, Sign, Delta)
    K1 = QCell*(1/(VCell/2));
    K2 = (1/(VCell/2))*(1/(Z*F));
    CCell = (K1*Delta*CTank + Sign*K2*Delta*It + CCellAnt)/(1+K1*Delta);
end

== matlab function MassTransfer/Liibrary block/Analitical/C4Tank/MATLAB Function ==
  data: Q input; CTank output; CCell input; CTankAnt input; VTank input; Delta input
function CTank = fcn(Q, CCell, CTankAnt, VTank, Delta)
    K3 = Q/VTank;
    CTank = (CCell*K3*Delta + CTankAnt)/(1+K3*Delta);
end

== matlab function MassTransfer/Liibrary block/Analitical/C5Cell/MATLAB Function ==
  data: QCell input; CCell output; CTank input; CCellAnt input; VCell input; It input; F input; Z input; Sign input; Delta input
function CCell = fcn(QCell, CTank, CCellAnt, VCell, It, F, Z, Sign, Delta)
    K1 = QCell*(1/(VCell/2));
    K2 = (1/(VCell/2))*(1/(Z*F));
    CCell = (K1*Delta*CTank + Sign*K2*Delta*It + CCellAnt)/(1+K1*Delta);
end

== matlab function MassTransfer/Liibrary block/Analitical/C5Tank/MATLAB Function ==
  data: Q input; CTank output; CCell input; CTankAnt input; VTank input; Delta input
function CTank = fcn(Q, CCell, CTankAnt, VTank, Delta)
    K3 = Q/VTank;
    CTank = (CCell*K3*Delta + CTankAnt)/(1+K3*Delta);
end

== matlab function MassTransfer/Liibrary block/Flow calculation anal/MATLAB Function ==
  data: C2 input; QCell output; C3 input; C4 input; C5 input; I input; F input
function QCell = fcn(C2, C3, C4, C5, I, F)
    if I > 0
        QCell = abs(I)/(F*(C2+C5)/2);
    else
        QCell = abs(I)/(F*(C3+C4)/2);
    end
end

== matlab function MassTransfer/Liibrary block/Flow calculation simulink/MATLAB Function ==
  data: C2 input; QCell output; C3 input; C4 input; C5 input; I input; F input
function QCell = fcn(C2, C3, C4, C5, I, F)
    if I > 0
        QCell = abs(I)/(F*(C2+C5)/2);
    else
        QCell = abs(I)/(F*(C3+C4)/2);
    end
end

== matlab function MassTransfer/QF tests1/Analitical/C2Cell/MATLAB Function ==
  data: QCell input; CCell output; CTank input; CCellAnt input; VCell input; It input; F input; Z input; Sign input; Delta input
function CCell = fcn(QCell, CTank, CCellAnt, VCell, It, F, Z, Sign, Delta)
    K1 = QCell*(1/(VCell/2));
    K2 = (1/(VCell/2))*(1/(Z*F));
    CCell = (K1*Delta*CTank + Sign*K2*Delta*It + CCellAnt)/(1+K1*Delta);
end

== matlab function MassTransfer/QF tests1/Analitical/C2Tank/MATLAB Function ==
  data: Q input; CTank output; CCell input; CTankAnt input; VTank input; Delta input
function CTank = fcn(Q, CCell, CTankAnt, VTank, Delta)
    K3 = Q/VTank;
    CTank = (CCell*K3*Delta + CTankAnt)/(1+K3*Delta);
end
